simulink model "publisher_task"  (Simulink 3.0)
undefined symbols (not defined in the file): Double, F64
libraries: genlib x4, mathlib x3, mqttlib x2, arclib x2, logiclib x1

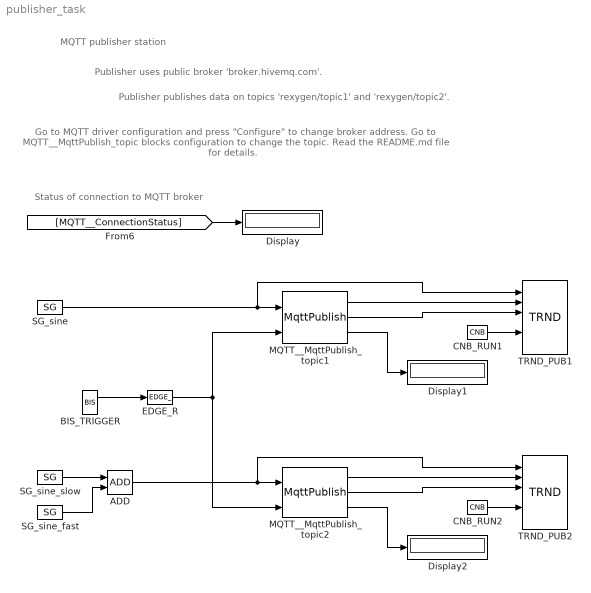
== system publisher_task ==
  note: MQTT publisher station
  note: Publisher publishes data on topics 'rexygen/topic1' and 'rexygen/topic2'.
  note: Publisher uses public broker 'broker.hivemq.com'.
  note: Status of connection to MQTT broker
  note: Go to MQTT driver configuration and press "Configure" to change broker address.
      | Go to MQTT__MqttPublish_topic blocks configuration to change the topic.
      |
      | Read the README.md file for details.
  ADD : mathlib/ADD
  BIS_TRIGGER : genlib/BIS  Y0=off  t1=1  t2=2  t3=5  t4=0  t5=0  t6=0  t7=0  t8=0  RPT=on
  CNB_RUN1 : mathlib/CNB  YCN=on
  CNB_RUN2 : mathlib/CNB  YCN=on
  Display : Display
      settings: Format=Best fit
  Display1 : Display
      settings: Format=Best fit
  Display2 : Display
      settings: Format=Best fit
  EDGE_R : logiclib/EDGE_  iedge=1: Rising edge
  MQTT__MqttPublish_topic1 : mqttlib/MqttPublish  topic=rexygen/topic1  QoS=1: QoS0 (At most once)  RETAIN=off  defBuffSize=80
  MQTT__MqttPublish_topic2 : mqttlib/MqttPublish  topic=rexygen/topic2  QoS=1: QoS0 (At most once)  RETAIN=off  defBuffSize=80
  SG_sine : genlib/SG  isig=1: SINE  amp=1  freq=0.02  phase=0  offset=0  ifrunit=1: Hz  iphunit=1: degrees
  SG_sine_fast : genlib/SG  isig=1: SINE  amp=3  freq=0.09  phase=0  ifrunit=1: Hz  iphunit=1: degrees  offset=0
  SG_sine_slow : genlib/SG  isig=1: SINE  amp=10  freq=0.025  phase=0  ifrunit=1: Hz  iphunit=1: degrees  offset=0
  TRND_PUB1 : arclib/TRND  n=4  l=1000  btype=8: Double (F64)  ptype1=1: Store  ptype2=1: Store  ptype3=1: Store  ptype4=1: Store  pfac=1  afac=0  arc=0  id=0  Title=MQTT publish topic 1  timesrc=1: CORETIMER
  TRND_PUB2 : arclib/TRND  n=4  l=1000  btype=8: Double (F64)  ptype1=1: Store  ptype2=1: Store  ptype3=1: Store  ptype4=1: Store  pfac=1  afac=0  arc=0  id=0  Title=MQTT publish topic 2  timesrc=1: CORETIMER
  wires:
  ADD/1 -> MQTT__MqttPublish_topic2/1, TRND_PUB2/1
  BIS_TRIGGER/1 -> EDGE_R/1
  CNB_RUN1/1 -> TRND_PUB1/5
  CNB_RUN2/1 -> TRND_PUB2/5
  EDGE_R/1 -> MQTT__MqttPublish_topic1/2, MQTT__MqttPublish_topic2/2
  [MQTT__ConnectionStatus] -> Display/1
  MQTT__MqttPublish_topic1/1 -> TRND_PUB1/2
  MQTT__MqttPublish_topic1/2 -> TRND_PUB1/3
  MQTT__MqttPublish_topic1/3 -> Display1/1
  MQTT__MqttPublish_topic2/1 -> TRND_PUB2/2
  MQTT__MqttPublish_topic2/2 -> TRND_PUB2/3
  MQTT__MqttPublish_topic2/3 -> Display2/1
  SG_sine/1 -> MQTT__MqttPublish_topic1/1, TRND_PUB1/1
  SG_sine_fast/1 -> ADD/2
  SG_sine_slow/1 -> ADD/1
